simulink model "dc_state_feedback2016"  (R2016a)
settings: Solver=VariableStepAuto  SolverMode=SingleTasking  StartTime=0.0  StopTime=10  RelTol=1e-3
values from neighbouring files (symbols this model uses):
  A = [0 1 0;0 -b/J K/J;0 -K/L -R/L]    [state_space_control.m]
  B = [0 ; 0 ; 1/L]    [state_space_control.m]
  C = [1  1  0]    [state_space_control.m]
  K1 = acker(A,B,[p1 p2 p3])    [state_space_control.m]
settings Model: Creator=asus  LastModifiedBy=asus
settings DataIOCC: ReturnWorkspaceOutputs=on
settings DebuggingCC: SFUnexpectedBacktrackingDiag=error  SFNoUnconditionalDefaultTransitionDiag=error
settings SFSimCC: SimUseLocalCustomCode=on
settings RTWCC: RTWUseLocalCustomCode=on
settings GRTTargetCC: TargetLangStandard=C99 (ISO)  GeneratePreprocessorConditionals=Use local settings
settings ConfigComp: CovMetricSettings=dwe  CovHtmlReporting=off  CovSaveCumulativeToWorkspaceVar=off  CovSaveSingleToWorkspaceVar=off  CovExternalEMLEnable=on

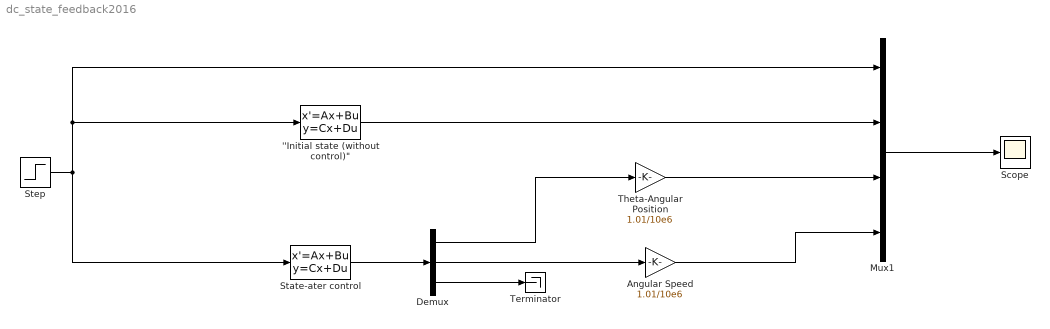
== system dc_state_feedback2016 ==
  "''Initial state (without control)\"" : StateSpace  A=A  B=B  C=C  D=0  X0=0
  Angular Speed : Gain  Gain=1.01/10e6
  Demux : Demux  Outputs=3
  Mux1 : Mux
  "Scope " : Scope
  State-ater control : StateSpace  A=A-B*K1  B=B  C=eye(3)  D=[0;0;0]  X0=0
  Step : Step  SampleTime=0
  Terminator : Terminator
  Theta-Angular Position : Gain  Gain=1.01/10e6
  wires:
  Mux1/1 -> "Scope "/1
  Step/1 -> State-ater control/1, Mux1/1, "''Initial state (without control)\""/1
  State-ater control/1 -> Demux/1
  Demux/3 -> Terminator/1
  Demux/1 -> Theta-Angular Position/1
  Theta-Angular Position/1 -> Mux1/3
  Demux/2 -> Angular Speed/1
  Angular Speed/1 -> Mux1/4
  "''Initial state (without control)\""/1 -> Mux1/2
